simulink model "APP_Chart"  (R2022b)
settings: Solver=FixedStepAuto  StartTime=0.0  StopTime=10.0  FixedStep=0.01  RelTol=1e-3
libraries: simulink x2
settings Model: Creator=MAAM  LastModifiedBy=MAAM

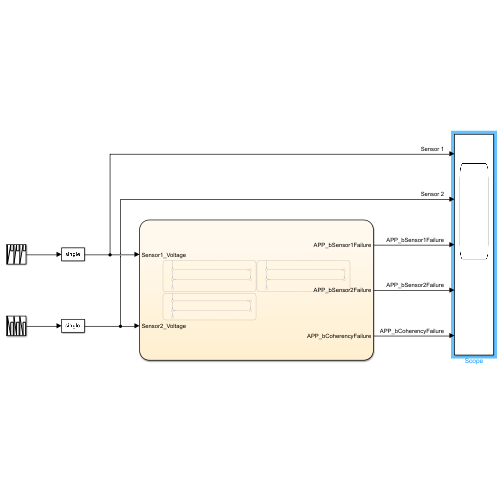
[thumbnail: Simulink's stored preview of the top-level diagram]
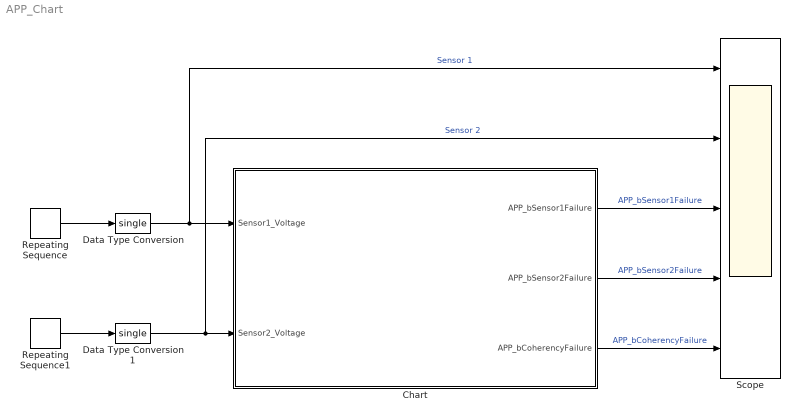
== system APP_Chart ==
  Chart : Stateflow chart  TreatAsAtomicUnit=on
  Data Type Conversion : DataTypeConversion  OutDataTypeStr=single  SaturateOnIntegerOverflow=off  RndMeth=Floor
  Data Type Conversion1 : DataTypeConversion  OutDataTypeStr=single  SaturateOnIntegerOverflow=off  RndMeth=Floor
  Repeating Sequence : simulink/Sources/Repeating Sequence  rep_seq_t=[0 1 1.001 6 6.001 10]  rep_seq_y=[5 5 0 5 3.5 3.5]
  Repeating Sequence1 : simulink/Sources/Repeating Sequence  rep_seq_t=[0 1 1.001 6 6.001 10]  rep_seq_y=[0 0 5 0 3.5 3.5]
  Scope : Scope  NumInputPorts=5
  wires:
  Chart/1(APP_bSensor1Failure) -> Scope/3  "APP_bSensor1Failure"
  Chart/3(APP_bCoherencyFailure) -> Scope/5  "APP_bCoherencyFailure"
  Chart/2(APP_bSensor2Failure) -> Scope/4  "APP_bSensor2Failure"
  Repeating Sequence/1 -> Data Type Conversion/1
  Repeating Sequence1/1 -> Data Type Conversion1/1
  Data Type Conversion/1 -> Scope/1, Chart/1(Sensor1_Voltage)  "Sensor 1"
  Data Type Conversion1/1 -> Scope/2, Chart/2(Sensor2_Voltage)  "Sensor 2"

== stateflow chart APP_Chart/Chart ==
  state Sensor1 [parallel]
    settings: executionOrder=1
    Sensor1 -> (junction 8)
    (junction 8) -> (junction 10) [order 1] : [(Sensor1_Voltage <= S_UpLim) && (Sensor1_Voltage >= S_LowLim)]
    (junction 8) -> (junction 38) [order 2] : {APP_bSensor1Failure = true;}
    (junction 10) -> (junction 18) : {APP_bSensor1Failure = false;}
    (junction 18) -> (junction 38)
    (junction 38) -> (junction 44)
  state Sensor2 [parallel]
    settings: executionOrder=3
    Sensor2 -> (junction 50)
    (junction 50) -> (junction 52) [order 1] : [(Sensor2_Voltage <= S_UpLim) && (Sensor2_Voltage >= S_LowLim)]
    (junction 50) -> (junction 53) [order 2] : {APP_bSensor2Failure = true;}
    (junction 52) -> (junction 55) : {APP_bSensor2Failure = false;}
    (junction 55) -> (junction 53)
    (junction 53) -> (junction 57)
  state coherency [parallel]
    settings: executionOrder=2
    coherency -> (junction 28)
    (junction 28) -> (junction 27) [order 1] : [((Sensor1_Voltage + Sensor2_Voltage) ~= S_Coherency)]
    (junction 28) -> (junction 41) [order 2] : {APP_bCoherencyFailure = false;}
    (junction 27) -> (junction 30) : {APP_bCoherencyFailure = true;}
    (junction 30) -> (junction 41)
    (junction 41) -> (junction 62)
  data: APP_bSensor1Failure output boolean; APP_bSensor2Failure output boolean; APP_bCoherencyFailure output boolean; Sensor1_Voltage input single; Sensor2_Voltage input single; S_LowLim constant single =0.5; S_UpLim constant single =4.5; S_Coherency constant single =5.0
